simulink model "A3_3_VorInvKin_23a"  (R2023a)
settings: Solver=FixedStepAuto  StartTime=0.0  StopTime=10  FixedStep=1e-3  RelTol=1e-3
values from neighbouring files (symbols this model uses):
  params = [l2 l3]    [A3_1_init_VorKin.m]    (also in A3_2_init_InvKin.m; init_InvKin.m)
settings Model: Creator=Flo  LastModifiedBy=Flo

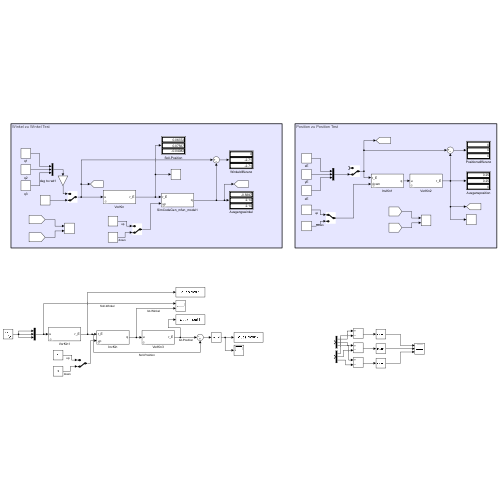
[thumbnail: Simulink's stored preview of the top-level diagram]
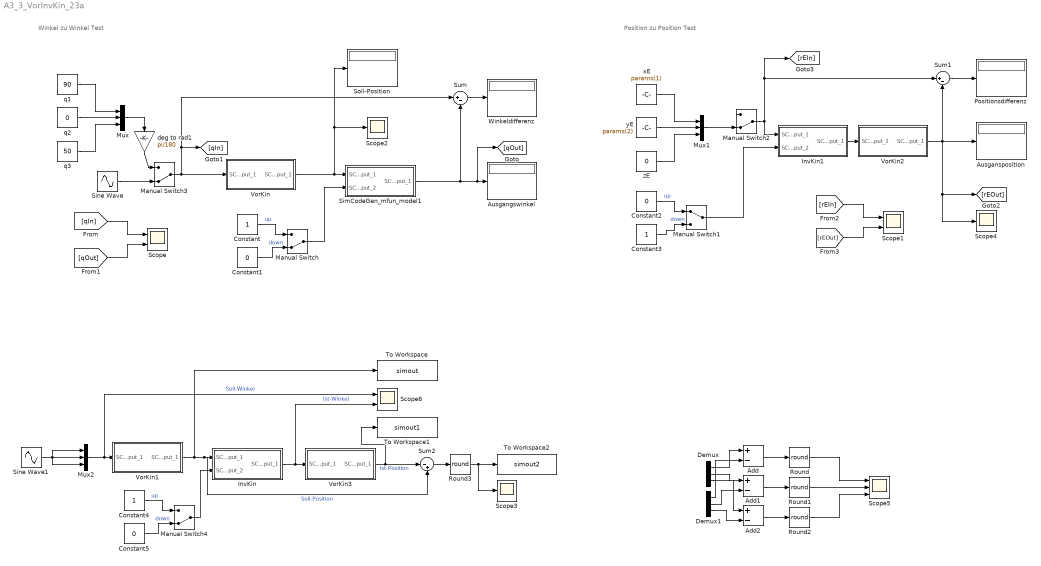
== system A3_3_VorInvKin_23a ==
  note: Winkel zu Winkel Test
  note: Position zu Position Test
  Add : Sum  Inputs=+-
  Add1 : Sum  Inputs=+-
  Add2 : Sum  Inputs=+-
  Ausgangswinkel : Display
  Ausgansposition : Display
  Constant : Constant
  Constant1 : Constant  Value=0
  Constant2 : Constant  Value=0
  Constant3 : Constant
  Constant4 : Constant
  Constant5 : Constant  Value=0
  Demux : Demux  Outputs=3
  Demux1 : Demux  Outputs=3
  InvKin : Subsystem  mask{SC_param_0=params}
      mask prompts: SC_param_0 "params"
      mask Display:
      | port_label('input', 1, 'r_E');
      | port_label('input', 2, 'up');
      | port_label('output', 1, 'q');
  InvKin1 : Subsystem  mask{SC_param_0=params}
      mask prompts: SC_param_0 "params"
      mask Display:
      | port_label('input', 1, 'r_E');
      | port_label('input', 2, 'down');
      | port_label('output', 1, 'q');
  Manual Switch{,2..4} (4 alike) : ManualSwitch  CurrentSetting=0
  Manual Switch1 : ManualSwitch
  Mux : Mux  Inputs=3
  Mux1 : Mux  Inputs=3
  Mux2 : Mux  Inputs=3
  Positionsdifferenz : Display
  Round{,1..3} (4 alike) : Rounding  Operator=round
  Scope : Scope  NumInputPorts=2
  Scope1 : Scope  NumInputPorts=2
  Scope2 : Scope
  Scope3 : Scope
  Scope4 : Scope
  Scope5 : Scope  NumInputPorts=3
  Scope6 : Scope  NumInputPorts=2
  SimCodeGen_mfun_model1 : Subsystem  mask{SC_param_0=params}
      mask prompts: SC_param_0 "params"
      mask Display:
      | port_label('input', 1, 'r_E');
      | port_label('input', 2, 'up');
      | port_label('output', 1, 'q');
  Sine Wave : Sin  Amplitude=60*pi/180  SampleTime=0  VectorParams1D=off
  Sine Wave1 : Sin  Amplitude=30*pi/180  SampleTime=0  VectorParams1D=off
  Soll-Position : Display
  Sum : Sum  Inputs=|+-
  Sum1 : Sum  Inputs=|+-
  Sum2 : Sum  Inputs=|-+
  To Workspace : ToWorkspace  VariableName=simout  SaveFormat=Timeseries  SampleTime=-1
  To Workspace1 : ToWorkspace  VariableName=simout1  SaveFormat=Timeseries  SampleTime=-1
  To Workspace2 : ToWorkspace  VariableName=simout2  SaveFormat=Timeseries  SampleTime=-1
  VorKin : Subsystem  mask{SC_param_0=params}
      mask prompts: SC_param_0 "params"
      mask Display:
      | port_label('input', 1, 'u');
      | port_label('output', 1, 'r_E');
  VorKin1 : Subsystem  mask{SC_param_0=params}
      mask prompts: SC_param_0 "params"
      mask Display:
      | port_label('input', 1, 'u');
      | port_label('output', 1, 'r_E');
  VorKin2 : Subsystem  mask{SC_param_0=params}
      mask prompts: SC_param_0 "params"
      mask Display:
      | port_label('input', 1, 'u');
      | port_label('output', 1, 'r_E');
  VorKin3 : Subsystem  mask{SC_param_0=params}
      mask prompts: SC_param_0 "params"
      mask Display:
      | port_label('input', 1, 'u');
      | port_label('output', 1, 'r_E');
  Winkeldifferenz : Display
  deg to rad1 : Gain  Gain=pi/180
  q1 : Constant  Value=90
  q2 : Constant  Value=0
  q3 : Constant  Value=50
  xE : Constant  Value=params(1)
  yE : Constant  Value=params(2)
  zE : Constant  Value=0
  wires:
  Constant/1 -> Manual Switch/1  "up"
  Constant1/1 -> Manual Switch/2  "down"
  Manual Switch/1 -> SimCodeGen_mfun_model1/2(SC_input_2)
  VorKin/1(SC_output_1) -> SimCodeGen_mfun_model1/1(SC_input_1), Scope2/1, Soll-Position/1
  SimCodeGen_mfun_model1/1(SC_output_1) -> [qOut], Ausgangswinkel/1, Sum/2
  q3/1 -> Mux/3
  q2/1 -> Mux/2
  q1/1 -> Mux/1
  Sum/1 -> Winkeldifferenz/1
  Manual Switch1/1 -> InvKin1/2(SC_input_2)
  Sum1/1 -> Positionsdifferenz/1
  Constant2/1 -> Manual Switch1/1  "up"
  VorKin2/1(SC_output_1) -> Scope4/1, [rEOut], Ausgansposition/1, Sum1/2
  zE/1 -> Mux1/3
  yE/1 -> Mux1/2
  Constant3/1 -> Manual Switch1/2  "down"
  xE/1 -> Mux1/1
  InvKin1/1(SC_output_1) -> VorKin2/1(SC_input_1)
  Mux1/1 -> Manual Switch2/2
  Manual Switch2/1 -> InvKin1/1(SC_input_1), [rEIn], Sum1/1
  Sine Wave/1 -> Manual Switch3/2
  [qIn] -> Scope/1
  [qOut] -> Scope/2
  [rEOut] -> Scope1/2
  [rEIn] -> Scope1/1
  Manual Switch3/1 -> VorKin/1(SC_input_1), [qIn], Sum/1
  Mux/1 -> deg to rad1/1
  deg to rad1/1 -> Manual Switch3/1
  VorKin1/1(SC_output_1) -> To Workspace/1, Sum2/2, InvKin/1(SC_input_1)  "Soll-Position"
  InvKin/1(SC_output_1) -> Scope6/2, VorKin3/1(SC_input_1)  "Ist-Winkel"
  VorKin3/1(SC_output_1) -> To Workspace1/1, Sum2/1  "Ist-Position"
  Constant5/1 -> Manual Switch4/2  "down"
  Constant4/1 -> Manual Switch4/1  "up"
  Manual Switch4/1 -> InvKin/2(SC_input_2)
  Mux2/1 -> Scope6/1, VorKin1/1(SC_input_1)  "Soll-Winkel"
  Sine Wave1/1 -> Mux2/3, Mux2/1, Mux2/2
  Demux1/3 -> Add2/2
  Demux/3 -> Add2/1
  Demux1/2 -> Add1/2
  Demux1/1 -> Add/2
  Demux/2 -> Add1/1
  Demux/1 -> Add/1
  Add/1 -> Round/1
  Round/1 -> Scope5/1
  Add2/1 -> Round2/1
  Add1/1 -> Round1/1
  Round1/1 -> Scope5/2
  Round2/1 -> Scope5/3
  Sum2/1 -> Round3/1
  Round3/1 -> Scope3/1, To Workspace2/1

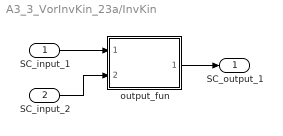
== system A3_3_VorInvKin_23a/InvKin ==
  SC_input_1 : Inport
  SC_input_2 : Inport  Port=2
  output_fun : MATLAB Function  TreatAsAtomicUnit=on
  SC_output_1 : Outport
  wires:
  output_fun/1(SC_output_0) -> SC_output_1/1
  SC_input_2/1 -> output_fun/2(SC_input_1)
  SC_input_1/1 -> output_fun/1(SC_input_0)

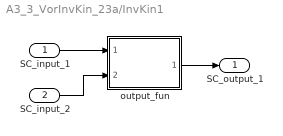
== system A3_3_VorInvKin_23a/InvKin1 ==
  SC_input_1 : Inport
  SC_input_2 : Inport  Port=2
  output_fun : MATLAB Function  TreatAsAtomicUnit=on
  SC_output_1 : Outport
  wires:
  SC_input_2/1 -> output_fun/2(SC_input_1)
  SC_input_1/1 -> output_fun/1(SC_input_0)
  output_fun/1(SC_output_0) -> SC_output_1/1

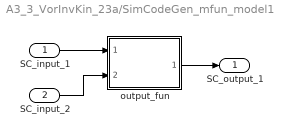
== system A3_3_VorInvKin_23a/SimCodeGen_mfun_model1 ==
  SC_input_1 : Inport
  SC_input_2 : Inport  Port=2
  output_fun : MATLAB Function  TreatAsAtomicUnit=on
  SC_output_1 : Outport
  wires:
  output_fun/1(SC_output_0) -> SC_output_1/1
  SC_input_2/1 -> output_fun/2(SC_input_1)
  SC_input_1/1 -> output_fun/1(SC_input_0)

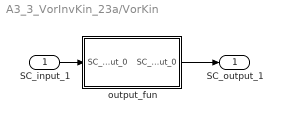
== system A3_3_VorInvKin_23a/VorKin ==
  SC_input_1 : Inport
  output_fun : MATLAB Function  TreatAsAtomicUnit=on
  SC_output_1 : Outport
  wires:
  SC_input_1/1 -> output_fun/1(SC_input_0)
  output_fun/1(SC_output_0) -> SC_output_1/1

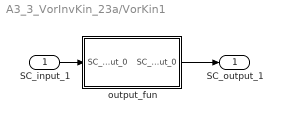
== system A3_3_VorInvKin_23a/VorKin1 ==
  SC_input_1 : Inport
  output_fun : MATLAB Function  TreatAsAtomicUnit=on
  SC_output_1 : Outport
  wires:
  SC_input_1/1 -> output_fun/1(SC_input_0)
  output_fun/1(SC_output_0) -> SC_output_1/1

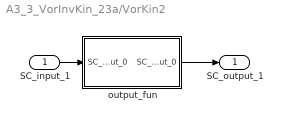
== system A3_3_VorInvKin_23a/VorKin2 ==
  SC_input_1 : Inport
  output_fun : MATLAB Function  TreatAsAtomicUnit=on
  SC_output_1 : Outport
  wires:
  SC_input_1/1 -> output_fun/1(SC_input_0)
  output_fun/1(SC_output_0) -> SC_output_1/1

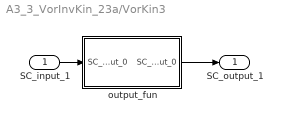
== system A3_3_VorInvKin_23a/VorKin3 ==
  SC_input_1 : Inport
  output_fun : MATLAB Function  TreatAsAtomicUnit=on
  SC_output_1 : Outport
  wires:
  SC_input_1/1 -> output_fun/1(SC_input_0)
  output_fun/1(SC_output_0) -> SC_output_1/1

== matlab function A3_3_VorInvKin_23a/VorKin/output_fun ==
  data: SC_input_0 input size=[3]; SC_output_0 output size=[3]; SC_param_0 parameter size=[2]
function SC_output_0  = y_fun(SC_input_0, SC_param_0)
    SC_output_0 = zeros(3,1);
    t1 = SC_input_0(1);
    t2 = cos(t1);
    t3 = SC_input_0(3);
    t4 = cos(t3);
    t5 = SC_param_0(2);
    t7 = SC_input_0(2);
    t8 = sin(t7);
    t9 = SC_param_0(1);
    t11 = t4 * t5 + t8 * t9;
    SC_output_0(1) = t11 * t2;
    t12 = sin(t3);
    t14 = cos(t7);
    SC_output_0(2) = t12 * t5 + t14 * t9;
    t16 = sin(t1);
    SC_output_0(3) = t16 * t11;
end

== matlab function A3_3_VorInvKin_23a/VorKin1/output_fun ==
  data: SC_input_0 input size=[3]; SC_output_0 output size=[3]; SC_param_0 parameter size=[2]
function SC_output_0  = y_fun(SC_input_0, SC_param_0)
    SC_output_0 = zeros(3,1);
    t1 = SC_input_0(1);
    t2 = cos(t1);
    t3 = SC_input_0(3);
    t4 = cos(t3);
    t5 = SC_param_0(2);
    t7 = SC_input_0(2);
    t8 = sin(t7);
    t9 = SC_param_0(1);
    t11 = t4 * t5 + t8 * t9;
    SC_output_0(1) = t11 * t2;
    t12 = sin(t3);
    t14 = cos(t7);
    SC_output_0(2) = t12 * t5 + t14 * t9;
    t16 = sin(t1);
    SC_output_0(3) = t16 * t11;
end

== matlab function A3_3_VorInvKin_23a/InvKin1/output_fun ==
  data: SC_input_0 input size=[3]; SC_output_0 output size=[3]; SC_input_1 input size=[1]; SC_param_0 parameter size=[2]
function SC_output_0  = y_fun(SC_input_0, SC_input_1, SC_param_0)
    SC_output_0 = zeros(3,1);
    SC_output_0(1) = atan2(SC_input_0(3), SC_input_0(1));
    if (SC_input_1(1) == 0)
      s1 = pi / 0.2e1 - atan2(SC_input_0(2), SC_input_0(1) / cos(atan2(SC_input_0(3), SC_input_0(1)))) - asin(SC_param_0(2) * (SC_input_0(1) ^ 2 + SC_input_0(2) ^ 2 + SC_input_0(3) ^ 2) ^ (-0.1e1 / 0.2e1) * sqrt(0.4e1 - (-SC_input_0(1) ^ 2 - SC_input_0(2) ^ 2 - SC_input_0(3) ^ 2 + SC_param_0(1) ^ 2 + SC_param_0(2) ^ 2) ^ 2 / SC_param_0(1) ^ 2 / SC_param_0(2) ^ 2) / 0.2e1);
    else
      s1 = pi / 0.2e1 - atan2(SC_input_0(2), SC_input_0(1) / cos(atan2(SC_input_0(3), SC_input_0(1)))) + asin(SC_param_0(2) * (SC_input_0(1) ^ 2 + SC_input_0(2) ^ 2 + SC_input_0(3) ^ 2) ^ (-0.1e1 / 0.2e1) * sqrt(0.4e1 - (-SC_input_0(1) ^ 2 - SC_input_0(2) ^ 2 - SC_input_0(3) ^ 2 + SC_param_0(1) ^ 2 + SC_param_0(2) ^ 2) ^ 2 / SC_param_0(1) ^ 2 / SC_param_0(2) ^ 2) / 0.2e1);
    end
    SC_output_0(2) = s1;
    if (SC_input_1(1) == 0)
      if (SC_input_1(1) == 0)
        s3 = pi / 0.2e1 - atan2(SC_input_0(2), SC_input_0(1) / cos(atan2(SC_input_0(3), SC_input_0(1)))) - asin(SC_param_0(2) * (SC_input_0(1) ^ 2 + SC_input_0(2) ^ 2 + SC_input_0(3) ^ 2) ^ (-0.1e1 / 0.2e1) * sqrt(0.4e1 - (-SC_input_0(1) ^ 2 - SC_input_0(2) ^ 2 - SC_input_0(3) ^ 2 + SC_param_0(1) ^ 2 + SC_param_0(2) ^ 2) ^ 2 / SC_param_0(1) ^ 2 / SC_param_0(2) ^ 2) / 0.2e1);
      else
        s3 = pi / 0.2e1 - atan2(SC_input_0(2), SC_input_0(1) / cos(atan2(SC_input_0(3), SC_input_0(1)))) + asin(SC_param_0(2) * (SC_input_0(1) ^ 2 + SC_input_0(2) ^ 2 + SC_input_0(3) ^ 2) ^ (-0.1e1 / 0.2e1) * sqrt(0.4e1 - (-SC_input_0(1) ^ 2 - SC_input_0(2) ^ 2 - SC_input_0(3) ^ 2 + SC_param_0(1) ^ 2 + SC_param_0(2) ^ 2) ^ 2 / SC_param_0(1) ^ 2 / SC_param_0(2) ^ 2) / 0.2e1);
      end
      s2 = -pi / 0.2e1 - s3 + acos((-SC_input_0(1) ^ 2 - SC_input_0(2) ^ 2 - SC_input_0(3) ^ 2 + SC_param_0(1) ^ 2 + SC_param_0(2) ^ 2) / SC_param_0(1) / SC_param_0(2) / 0.2e1);
    else
      if (SC_input_1(1) == 0)
        s4 = pi / 0.2e1 - atan2(SC_input_0(2), SC_input_0(1) / cos(atan2(SC_input_0(3), SC_input_0(1)))) - asin(SC_param_0(2) * (SC_input_0(1) ^ 2 + SC_input_0(2) ^ 2 + SC_input_0(3) ^ 2) ^ (-0.1e1 / 0.2e1) * sqrt(0.4e1 - (-SC_input_0(1) ^ 2 - SC_input_0(2) ^ 2 - SC_input_0(3) ^ 2 + SC_param_0(1) ^ 2 + SC_param_0(2) ^ 2) ^ 2 / SC_param_0(1) ^ 2 / SC_param_0(2) ^ 2) / 0.2e1);
      else
        s4 = pi / 0.2e1 - atan2(SC_input_0(2), SC_input_0(1) / cos(atan2(SC_input_0(3), SC_input_0(1)))) + asin(SC_param_0(2) * (SC_input_0(1) ^ 2 + SC_input_0(2) ^ 2 + SC_input_0(3) ^ 2) ^ (-0.1e1 / 0.2e1) * sqrt(0.4e1 - (-SC_input_0(1) ^ 2 - SC_input_0(2) ^ 2 - SC_input_0(3) ^ 2 + SC_param_0(1) ^ 2 + SC_param_0(2) ^ 2) ^ 2 / SC_param_0(1) ^ 2 / SC_param_0(2) ^ 2) / 0.2e1);
      end
      s2 = 0.3e1 / 0.2e1 * pi - s4 - acos((-SC_input_0(1) ^ 2 - SC_input_0(2) ^ 2 - SC_input_0(3) ^ 2 + SC_param_0(1) ^ 2 + SC_param_0(2) ^ 2) / SC_param_0(1) / SC_param_0(2) / 0.2e1);
    end
    SC_output_0(3) = s2;
end

== matlab function A3_3_VorInvKin_23a/VorKin2/output_fun ==
  data: SC_input_0 input size=[3]; SC_output_0 output size=[3]; SC_param_0 parameter size=[2]
function SC_output_0  = y_fun(SC_input_0, SC_param_0)
    SC_output_0 = zeros(3,1);
    t1 = SC_input_0(1);
    t2 = cos(t1);
    t3 = SC_input_0(3);
    t4 = cos(t3);
    t5 = SC_param_0(2);
    t7 = SC_input_0(2);
    t8 = sin(t7);
    t9 = SC_param_0(1);
    t11 = t4 * t5 + t8 * t9;
    SC_output_0(1) = t11 * t2;
    t12 = sin(t3);
    t14 = cos(t7);
    SC_output_0(2) = t12 * t5 + t14 * t9;
    t16 = sin(t1);
    SC_output_0(3) = t16 * t11;
end

== matlab function A3_3_VorInvKin_23a/InvKin/output_fun ==
  data: SC_input_0 input size=[3]; SC_output_0 output size=[3]; SC_input_1 input size=[1]; SC_param_0 parameter size=[2]
function SC_output_0  = y_fun(SC_input_0, SC_input_1, SC_param_0)
    SC_output_0 = zeros(3,1);
    t1 = SC_input_0(3);
    t2 = SC_input_0(1);
    SC_output_0(1) = atan2(t1, t2);
    t4 = SC_input_0(2);
    t5 = t2 ^ 2;
    t6 = t1 ^ 2;
    t8 = sqrt(t5 + t6);
    t9 = atan2(t4, t8);
    t10 = SC_param_0(2);
    t11 = t4 ^ 2;
    t13 = sqrt(t5 + t11 + t6);
    t16 = SC_param_0(1);
    t17 = t16 ^ 2;
    t18 = t10 ^ 2;
    t19 = -t5 - t11 - t6 + t17 + t18;
    t20 = t19 ^ 2;
    t26 = sqrt(0.4e1 - 0.1e1 / t18 / t17 * t20);
    t29 = asin(t26 / t13 * t10 / 0.2e1);
    t31 = (-1) ^ SC_input_1(1);
    t32 = t31 * t29;
    SC_output_0(2) = pi / 0.2e1 - t9 + t32;
    t38 = acos(0.1e1 / t10 / t16 * t19 / 0.2e1);
    SC_output_0(3) = t9 - t32 + t31 * (pi - t38);
end

== matlab function A3_3_VorInvKin_23a/VorKin3/output_fun ==
  data: SC_input_0 input size=[3]; SC_output_0 output size=[3]; SC_param_0 parameter size=[2]
function SC_output_0  = y_fun(SC_input_0, SC_param_0)
    SC_output_0 = zeros(3,1);
    t1 = SC_input_0(1);
    t2 = cos(t1);
    t3 = SC_input_0(3);
    t4 = cos(t3);
    t5 = SC_param_0(2);
    t7 = SC_input_0(2);
    t8 = sin(t7);
    t9 = SC_param_0(1);
    t11 = t4 * t5 + t8 * t9;
    SC_output_0(1) = t11 * t2;
    t12 = sin(t3);
    t14 = cos(t7);
    SC_output_0(2) = t12 * t5 + t14 * t9;
    t16 = sin(t1);
    SC_output_0(3) = t16 * t11;
end

== matlab function A3_3_VorInvKin_23a/SimCodeGen_mfun_model1/output_fun ==
  data: SC_input_0 input size=[3]; SC_output_0 output size=[3]; SC_input_1 input size=[1]; SC_param_0 parameter size=[2]
function SC_output_0  = y_fun(SC_input_0, SC_input_1, SC_param_0)
    SC_output_0 = zeros(3,1);
    t1 = SC_input_0(3);
    t2 = SC_input_0(1);
    SC_output_0(1) = atan2(t1, t2);
    t4 = SC_input_0(2);
    t5 = t2 ^ 2;
    t6 = t1 ^ 2;
    t8 = sqrt(t5 + t6);
    t9 = atan2(t4, t8);
    t10 = SC_param_0(2);
    t11 = t4 ^ 2;
    t13 = sqrt(t5 + t11 + t6);
    t16 = SC_param_0(1);
    t17 = t16 ^ 2;
    t18 = t10 ^ 2;
    t19 = -t5 - t11 - t6 + t17 + t18;
    t20 = t19 ^ 2;
    t26 = sqrt(0.4e1 - 0.1e1 / t18 / t17 * t20);
    t29 = asin(t26 / t13 * t10 / 0.2e1);
    t31 = (-1) ^ SC_input_1(1);
    t32 = t31 * t29;
    SC_output_0(2) = pi / 0.2e1 - t9 + t32;
    t38 = acos(0.1e1 / t10 / t16 * t19 / 0.2e1);
    SC_output_0(3) = t9 - t32 + t31 * (pi - t38);
end
